simulink model "Car_dynamics_model"  (R2024a)
settings: Solver=VariableStepAuto  StartTime=0.0  StopTime=40  RelTol=1e-3
values from neighbouring files (symbols this model uses):
  C = 2.45    [test3_pace_jka.m]    (also in test3_simulink.m = 0.55)
  force_scaling = 2000    [test3_simulink.m]
  m = 1200    [test3_simulink.m]
  Re = 0.01    [test3_simulink.m]
  Rw = 0.001*(17*25.4+215*0.55*2)/2    (= 0.33415)    [test3_simulink.m]
libraries: SignalEditorBlockLib x1
settings Model: Creator=Corey  LastModifiedBy=Corey

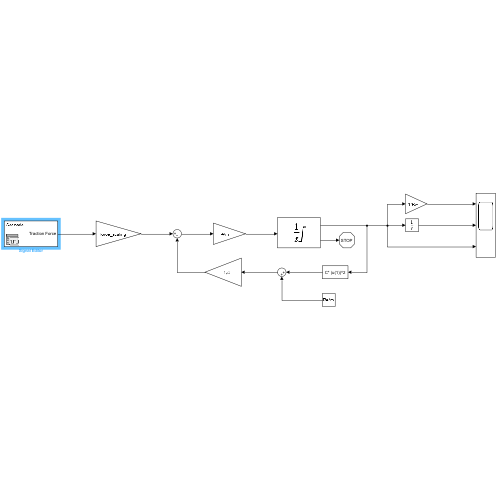
[thumbnail: Simulink's stored preview of the top-level diagram]
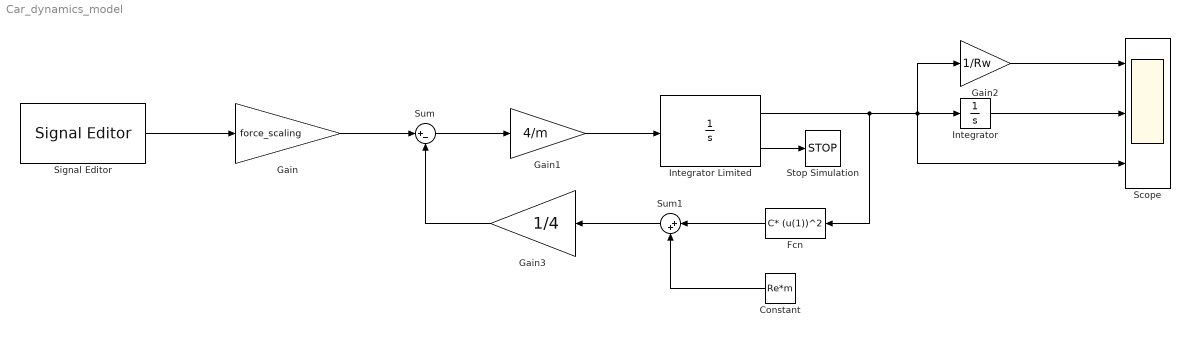
== system Car_dynamics_model ==
  Constant : Constant  Value=Re*m
  Fcn : Fcn  Expr=C* (u(1))^2
  Gain : Gain  Gain=force_scaling
  Gain1 : Gain  Gain=4/m
  Gain2 : Gain  Gain=1/Rw
  Gain3 : Gain  Gain=1/4
  Integrator : Integrator
  Integrator Limited : Integrator  InitialCondition=10  LimitOutput=on  UpperSaturationLimit=Inf  LowerSaturationLimit=0  ShowSaturationPort=on
  Scope : Scope  NumInputPorts=3
  Signal Editor : SignalEditorBlockLib/Signal Editor  FileName=Traction_Force.mat  ActiveScenario=Scenario  ActiveSignal=Traction Force  IsBus=off  OutputBusObjectStr=Bus: BusObject  SampleTime=0  Interpolate=off  ZeroCross=off  OutputAfterFinalValue=Setting to zero  Unit=inherit  PreserveSignalName=on  ApplySigPropsToAllScenarios=on  ApplySigPropsToAllSignals=off
  Stop Simulation : Stop
  Sum : Sum  Inputs=|+-
  Sum1 : Sum  Inputs=|++
  wires:
  Signal Editor/1 -> Gain/1
  Gain/1 -> Sum/1
  Sum/1 -> Gain1/1
  Gain1/1 -> Integrator Limited/1
  Integrator Limited/2 -> Stop Simulation/1
  Integrator Limited/1 -> Fcn/1, Scope/3, Gain2/1, Integrator/1
  Gain2/1 -> Scope/1
  Integrator/1 -> Scope/2
  Fcn/1 -> Sum1/1
  Constant/1 -> Sum1/2
  Sum1/1 -> Gain3/1
  Gain3/1 -> Sum/2
